simulink model "pmsm_foc"  (R2021a)
settings: Solver=ode23t  StartTime=0.0  StopTime=1  FixedStep=0.000001  RelTol=1e-3
model workspace (MAT data in the model file):
  G1 = -4000
  G2 = 14000
  L = 0.00395
  Rs = 0.485
  Ts = 1e-06
  a = Simulink.Parameter
  a.DataType = 'auto'
  a.Dimensions = [0 0]
undefined symbols (not defined in the file or in its folder): DiscIntNeverNeededParam
libraries: pid_lib x3, spsDCVoltageSourceLib x1, spsGroundLib x1, spsPermanentMagnetSynchronousMachineLib x1, simulink x1, spsUniversalBridgeLib x1, spspowerguiLib x1
settings Model: OrderedModelArguments=off  Creator=SkyLin  LastModifiedBy=SkyLin
settings OptimizationCC: GainParamInheritBuiltInType=on  UseFloatMulNetSlope=on
settings RTWCC: GenCodeOnly=on

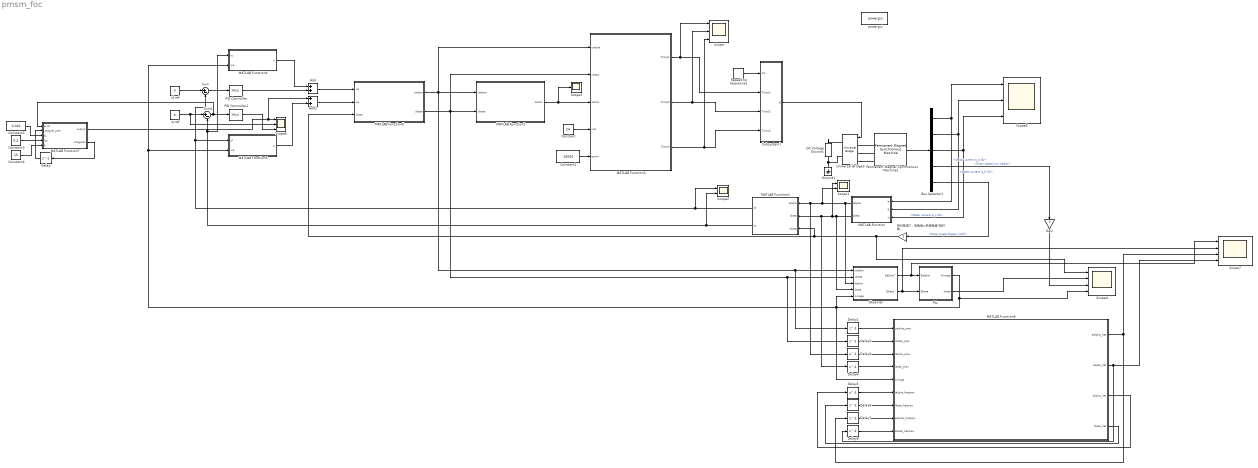
== system pmsm_foc ==
  Add : Sum
  Add1 : Sum
  Bus Selector1 : BusSelector  OutputSignals=Stator current is_a (A),Stator current is_b (A),Stator current is_c (A),Rotor speed wm (rad/s),Rotor angle thetam (rad)
  Constant : Constant  Value=24
  Constant1 : Constant  Value=10000
  Constant2 : Constant  Value=0.001
  Constant3 : Constant  Value=0.4
  Constant4 : Constant  Value=15
  DC Voltage Source1 : spsDCVoltageSourceLib/DC Voltage Source  Amplitude=24  Measurements=None
  Delay{,1..8} (9 alike) : Delay  DelayLength=1
  Gain : Gain  Gain=7
  Ground1 : spsGroundLib/Ground  LConnTagsString=a
  MATLAB Function : MATLAB Function  TreatAsAtomicUnit=on
  MATLAB Function1 : MATLAB Function  TreatAsAtomicUnit=on
  MATLAB Function2 : MATLAB Function  TreatAsAtomicUnit=on
  MATLAB Function3 : MATLAB Function  TreatAsAtomicUnit=on
  MATLAB Function4 : MATLAB Function  TreatAsAtomicUnit=on
  MATLAB Function5 : MATLAB Function  TreatAsAtomicUnit=on
  MATLAB Function6 : MATLAB Function  TreatAsAtomicUnit=on
  MATLAB Function7 : MATLAB Function  TreatAsAtomicUnit=on
  MATLAB Function8 : MATLAB Function  TreatAsAtomicUnit=on
  Observer : Subsystem
  PID Controller : pid_lib/PID Controller  Controller=PI  Form=Parallel  TimeDomain=Discrete-time  UseExternalTs=off  SampleTime=-1  IntegratorMethod=Forward Euler  FilterMethod=Forward Euler  ControllerParametersSource=internal  P=3.05  I=374.17  D=0  UseFilter=on  N=100  TunerSelectOption=Transfer Function Based (PID Tuner App)  InitialConditionSource=internal  InitialConditionForIntegrator=0  InitialConditionForFilter=0  DifferentiatorICPrevScaledInput=0  ExternalReset=none  TrackingMode=off  Kt=1  LimitOutput=on  SatLimitsSource=internal  UpperSaturationLimit=24  LowerSaturationLimit=-24  LinearizeAsGain=on  AntiWindupMode=none  Kb=1  POutMin=[]  POutMax=[]  IOutMin=[]  IOutMax=[]  DOutMin=[]  DOutMax=[]  NOutMin=[]  NOutMax=[]  SumOutMin=[]  SumOutMax=[]  SaturationOutMin=[]  SaturationOutMax=[]  PParamMin=[]  PParamMax=[]  IParamMin=[]  IParamMax=[]  DParamMin=[]  DParamMax=[]  NParamMin=[]  NParamMax=[]  KbParamMin=[]  KbParamMax=[]  KtParamMin=[]  KtParamMax=[]  KbOutMin=[]  KbOutMax=[]  KtOutMin=[]  KtOutMax=[]  IntegratorOutMin=[]  IntegratorOutMax=[]  FilterOutMin=[]  FilterOutMax=[]  SumI1OutMin=[]  SumI1OutMax=[]  SumI2OutMin=[]  SumI2OutMax=[]  SumI3OutMin=[]  SumI3OutMax=[]  SumI4OutMin=[]  SumI4OutMax=[]  SumDOutMin=[]  SumDOutMax=[]  DifferentiatorOutMin=[]  DifferentiatorOutMax=[]  FilterDiffOutCoefMin=[]  FilterDiffOutCoefMax=[]  ReciprocalOutMin=[]  ReciprocalOutMax=[]  SumDenOutMin=[]  SumDenOutMax=[]  SumNumOutMin=[]  SumNumOutMax=[]  DivideOutMin=[]  DivideOutMax=[]  UdiffTsProdOutMin=[]  UdiffTsProdOutMax=[]  NTsProdOutMin=[]  NTsProdOutMax=[]  UintegralTsProdOutMin=[]  UintegralTsProdOutMax=[]  UngainTsProdOutMin=[]  UngainTsProdOutMax=[]  IntegratorContinuousStateAttributes=''  IntegratorStateMustResolveToSignalObject=off  IntegratorRTWStateStorageClass=Auto  FilterContinuousStateAttributes=''  FilterStateMustResolveToSignalObject=off  FilterRTWStateStorageClass=Auto  ParallelPVariant=InternalParameters  IdealPVariant=Disabled  IVariant=InternalParameters  DVariant=Disabled  IntegratorVariant=Discrete  SatVariant=Enabled  AWVariant=Passthrough  PCopyVariant=Disabled  TRVariant=Disabled  FdbkBlocksVariant=Forward  IdealPFdbkVariant=Disabled  SatFdbkVariant=Disabled  DerivativeFilterVariant=Disabled  NVariant=Disabled  NCopyVariant=Disabled_SignalSpec  FilterICVariant=Disabled  IntegratorICVariant=InternalICs  ExternalResetVariant=Disabled  TRSumVariant=Passthrough  SumFdbkVariant=Disabled  SumVariant=Sum_PI  TsampFilterVariant=InternalTs  TsampNgainVariant=Passthrough  TsampIntegralVariant=Passthrough  ExternalSaturationOutDataTypeStr=Inherit: Same as second input
  PID Controller1 : pid_lib/PID Controller  Controller=PI  Form=Parallel  TimeDomain=Discrete-time  UseExternalTs=off  SampleTime=-1  IntegratorMethod=Forward Euler  FilterMethod=Forward Euler  ControllerParametersSource=internal  P=3.15  I=374.17  D=0  UseFilter=on  N=100  TunerSelectOption=Transfer Function Based (PID Tuner App)  InitialConditionSource=internal  InitialConditionForIntegrator=0  InitialConditionForFilter=0  DifferentiatorICPrevScaledInput=0  ExternalReset=none  TrackingMode=off  Kt=1  LimitOutput=on  SatLimitsSource=internal  UpperSaturationLimit=24  LowerSaturationLimit=-24  LinearizeAsGain=on  AntiWindupMode=none  Kb=1  POutMin=[]  POutMax=[]  IOutMin=[]  IOutMax=[]  DOutMin=[]  DOutMax=[]  NOutMin=[]  NOutMax=[]  SumOutMin=[]  SumOutMax=[]  SaturationOutMin=[]  SaturationOutMax=[]  PParamMin=[]  PParamMax=[]  IParamMin=[]  IParamMax=[]  DParamMin=[]  DParamMax=[]  NParamMin=[]  NParamMax=[]  KbParamMin=[]  KbParamMax=[]  KtParamMin=[]  KtParamMax=[]  KbOutMin=[]  KbOutMax=[]  KtOutMin=[]  KtOutMax=[]  IntegratorOutMin=[]  IntegratorOutMax=[]  FilterOutMin=[]  FilterOutMax=[]  SumI1OutMin=[]  SumI1OutMax=[]  SumI2OutMin=[]  SumI2OutMax=[]  SumI3OutMin=[]  SumI3OutMax=[]  SumI4OutMin=[]  SumI4OutMax=[]  SumDOutMin=[]  SumDOutMax=[]  DifferentiatorOutMin=[]  DifferentiatorOutMax=[]  FilterDiffOutCoefMin=[]  FilterDiffOutCoefMax=[]  ReciprocalOutMin=[]  ReciprocalOutMax=[]  SumDenOutMin=[]  SumDenOutMax=[]  SumNumOutMin=[]  SumNumOutMax=[]  DivideOutMin=[]  DivideOutMax=[]  UdiffTsProdOutMin=[]  UdiffTsProdOutMax=[]  NTsProdOutMin=[]  NTsProdOutMax=[]  UintegralTsProdOutMin=[]  UintegralTsProdOutMax=[]  UngainTsProdOutMin=[]  UngainTsProdOutMax=[]  IntegratorContinuousStateAttributes=''  IntegratorStateMustResolveToSignalObject=off  IntegratorRTWStateStorageClass=Auto  FilterContinuousStateAttributes=''  FilterStateMustResolveToSignalObject=off  FilterRTWStateStorageClass=Auto  ParallelPVariant=InternalParameters  IdealPVariant=Disabled  IVariant=InternalParameters  DVariant=Disabled  IntegratorVariant=Discrete  SatVariant=Enabled  AWVariant=Passthrough  PCopyVariant=Disabled  TRVariant=Disabled  FdbkBlocksVariant=Forward  IdealPFdbkVariant=Disabled  SatFdbkVariant=Disabled  DerivativeFilterVariant=Disabled  NVariant=Disabled  NCopyVariant=Disabled_SignalSpec  FilterICVariant=Disabled  IntegratorICVariant=InternalICs  ExternalResetVariant=Disabled  TRSumVariant=Passthrough  SumFdbkVariant=Disabled  SumVariant=Sum_PI  TsampFilterVariant=InternalTs  TsampNgainVariant=Passthrough  TsampIntegralVariant=Passthrough  ExternalSaturationOutDataTypeStr=Inherit: Same as second input
  PLL : Subsystem
  Permanent Magnet Synchronous Machine1 : spsPermanentMagnetSynchronousMachineLib/Permanent Magnet Synchronous Machine  NbPhases=3  FluxDistribution=Sinusoidal  RotorType=Round  MechanicalLoad=Torque Tm  PresetModel=No  ShowDetailedParameters=on  MeasurementBus=off  Resistance=0.485  Inductance=8.5e-3  dqInductances=[8.5e-3,8.5e-3]  La=0.00395  MachineConstant=Flux linkage established by magnets (V.s)  Flux=0.0041087  VoltageCst=5.2167  TorqueCst=0.043141  Flat=120  Mechanical=[0.00007 0.04924 7 0]  PolePairs=4  InitialConditions=[0,0, 0,0]  InitialConditions5ph=[0 0 0 0 0 0]  RefAngle=Aligned with phase A axis (original Park)  IterativeDiscreteModel=Trapezoidal non iterative  TsBlock=-1  TsPowergui=0
  Repeating Sequence1 : simulink/Sources/Repeating Sequence  rep_seq_t=[0 0.0001 0.0002]  rep_seq_y=[0 10000 0]
  Scope : Scope  NumInputPorts=3
  Scope1 : Scope  NumInputPorts=2
  Scope2 : Scope  NumInputPorts=2
  Scope3 : Scope
  Scope4 : Scope  NumInputPorts=4
  Scope5 : Scope  NumInputPorts=3
  Scope6 : Scope  NumInputPorts=3
  Scope7 : Scope  NumInputPorts=4
  Subsystem1 : Subsystem
  Sum : Sum  Inputs=|+-
  Sum1 : Sum  Inputs=|+-
  Universal Bridge3 : spsUniversalBridgeLib/Universal Bridge  Arms=3  SnubberResistance=1e5  SnubberCapacitance=inf  Device=MOSFET / Diodes  Ron=1e-3  Lon=0  ForwardVoltages="[  0  0  ]"  ForwardVoltage=0  GTOparameters=[ 10e-6 , 20e-6 ]  IGBTparameters=[ 1e-6 , 2e-6 ]  Measurements=None  Measurements_2=None  converterType=Rectifier
  id ref : Constant  Value=0
  iq ref : Constant  Value=4
  powergui : spspowerguiLib/powergui  Priority=1  SimulationMode=Discrete  SampleTime=10E-6  frequency=60  Iterations=50  frequencyindice=0  Pbase=100e6  ErrMax=1e-4  UnitsV=kV  UnitsW=MW  buscounter=0  FunctionMessages=off  echomessages=off  EnableUseOfTLC=off  CurrentSourceSwitches=off  DisableSnubberDevices=off  DisableRonSwitches=off  DisableVfSwitches=off  DisplayEquations=off  AutomaticDiscreteSolvers=off  SolverType=Tustin/Backward Euler (TBE)  Interpol=off  ExternalGateDelay=off  methode=off  Ts=100  x0status=blocks  SPID=on  SwTol=0  HookPort=off  NonlinearTolerance=1e-4  nMaxIteration=100  ContinueOnMaxIteration=off  RestoreLinks=warning  ResistiveCurrentMeasurement=off  Frange=[0:2:500]  Ylog=off  Xlog=on  ShowGrid=off  save=off  variable=ZData  structure=0  ZoomFFT=off  StartTime=0.0  cycles=1  DisplayStyle=1  fundamental=60  FreqAxis=off  MaxFrequency=1000  frequencyindicesteady=1  RmsSteady=1  display=off
  极对数是7，电角度=机械角度*极对数 : Gain  Gain=7
  wires:
  Repeating Sequence1/1 -> Subsystem1/1(In1)
  Subsystem1/1(g) -> Universal Bridge3/1
  Permanent Magnet Synchronous Machine1/1 -> Bus Selector1/1
  Bus Selector1/1 -> MATLAB Function/1(ia), Scope5/1  "<Stator current is_a (A)>"
  Bus Selector1/2 -> Scope5/2, MATLAB Function/2(ib)  "<Stator current is_b (A)>"
  Bus Selector1/3 -> Scope5/3, MATLAB Function/3(ic)  "<Stator current is_c (A)>"
  极对数是7，电角度=机械角度*极对数/1 -> Scope4/1, MATLAB Function1/3(theta), MATLAB Function6/3(theta)
  MATLAB Function/1(ialpha) -> Observer/3(ialpha), Scope1/2, Delay3/1, MATLAB Function1/1(ialpha)
  MATLAB Function/2(ibeta) -> Scope1/1, Delay4/1, MATLAB Function1/2(ibeta), Observer/4(ibeta)
  MATLAB Function6/1(ualpha) -> MATLAB Function3/1(ualpha), Delay1/1, Observer/1(ualpha), MATLAB Function2/1(ualpha)
  MATLAB Function6/2(ubeta) -> MATLAB Function3/2(ubeta), MATLAB Function2/2(ubeta), Delay2/1, Observer/2(ubeta)
  MATLAB Function2/1(sector) -> Scope3/1, MATLAB Function3/3(sector)
  Constant/1 -> MATLAB Function3/4(udc)
  Constant1/1 -> MATLAB Function3/5(tpwm)
  MATLAB Function3/1(Tcmp1) -> Scope/1, Subsystem1/2(Tcmp1)
  MATLAB Function3/2(Tcmp2) -> Scope/2, Subsystem1/3(Tcmp2)
  MATLAB Function3/3(Tcmp3) -> Scope/3, Subsystem1/4(Tcmp3)
  Bus Selector1/5 -> 极对数是7，电角度=机械角度*极对数/1  "<Rotor angle thetam (rad)>"
  Observer/1(Ealpha^) -> Scope7/1, PLL/1(Ealpha)
  Observer/2(Ebeta^) -> PLL/2(Ebeta), Scope7/2
  id ref/1 -> Sum/1
  MATLAB Function1/1(id) -> Scope2/1, MATLAB Function5/1(id), Sum/2
  iq ref/1 -> Scope6/2, Sum1/1
  Sum/1 -> PID Controller/1
  Sum1/1 -> MATLAB Function7/1(error), PID Controller1/1
  MATLAB Function1/2(iq) -> Scope2/2, MATLAB Function4/1(iq), Sum1/2
  Bus Selector1/4 -> Gain/1  "<Rotor speed wm (rad/s)>"
  MATLAB Function4/1(y) -> Add/1
  PID Controller/1 -> Add/2
  Add/1 -> MATLAB Function6/1(ud)
  Add1/1 -> MATLAB Function6/2(uq)
  PID Controller1/1 -> Scope6/3
  MATLAB Function5/1(y) -> Add1/2
  PLL/2(theta) -> Scope4/2
  Gain/1 -> Scope4/3
  PLL/1(Omega) -> MATLAB Function8/5(omega), MATLAB Function4/2(we), MATLAB Function5/2(we), Observer/5(omega), Scope4/4
  Constant2/1 -> MATLAB Function7/3(ts)
  MATLAB Function7/1(output) -> Add1/1, Scope6/1
  MATLAB Function7/2(integeral) -> Delay/1
  Delay/1 -> MATLAB Function7/2(integral_prev)
  Constant3/1 -> MATLAB Function7/4(kp)
  Constant4/1 -> MATLAB Function7/5(ki)
  Delay1/1 -> MATLAB Function8/1(ualpha_prev)
  Delay2/1 -> MATLAB Function8/2(ubeta_prev)
  Delay3/1 -> MATLAB Function8/3(ialpha_prev)
  Delay4/1 -> MATLAB Function8/4(ibeta_prev)
  Delay5/1 -> MATLAB Function8/6(ialpha_hatprev)
  Delay6/1 -> MATLAB Function8/7(ibeta_hatprev)
  Delay7/1 -> MATLAB Function8/8(ealpha_hatprev)
  Delay8/1 -> MATLAB Function8/9(ebeta_hatprev)
  MATLAB Function8/3(ialpha_hat) -> Delay5/1
  MATLAB Function8/4(ibeta_hat) -> Delay6/1
  MATLAB Function8/2(ebeta_hat) -> Delay8/1, Scope7/4
  MATLAB Function8/1(ealpha_hat) -> Delay7/1, Scope7/3
  connections:
  DC Voltage Source1/RConn1 -- Universal Bridge3/RConn1
  Permanent Magnet Synchronous Machine1/LConn1 -- Universal Bridge3/LConn1
  Universal Bridge3/LConn2 -- Permanent Magnet Synchronous Machine1/LConn2
  Universal Bridge3/LConn3 -- Permanent Magnet Synchronous Machine1/LConn3
  DC Voltage Source1/LConn1 -- Ground1/LConn1 -- Universal Bridge3/RConn2

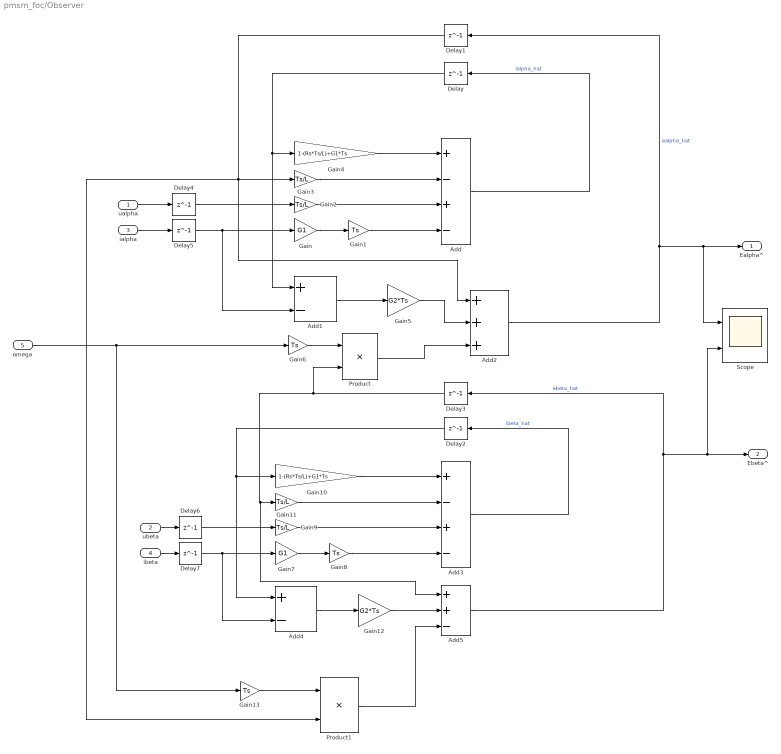
== system pmsm_foc/Observer ==
  ualpha : Inport
  ubeta : Inport  Port=2
  ialpha : Inport  Port=3
  ibeta : Inport  Port=4
  omega : Inport  Port=5
  Add : Sum  Inputs=+-+-
  Add1 : Sum  Inputs=+-
  Add2 : Sum  Inputs=+++
  Add3 : Sum  Inputs=+-+-
  Add4 : Sum  Inputs=+-
  Add5 : Sum  Inputs=++-
  Delay{,1..7} (8 alike) : Delay  DelayLength=1
  Gain : Gain  Gain=G1
  Gain{1,6,8,13} (4 alike) : Gain  Gain=Ts
  Gain10 : Gain  Gain=1-(Rs*Ts/L)+G1*Ts
  Gain{2..3,9,11} (4 alike) : Gain  Gain=Ts/L
  Gain12 : Gain  Gain=G2*Ts
  Gain4 : Gain  Gain=1-(Rs*Ts/L)+G1*Ts
  Gain5 : Gain  Gain=G2*Ts
  Gain7 : Gain  Gain=G1
  Product : Product
  Product1 : Product
  Scope : Scope  NumInputPorts=2
  Ealpha^ : Outport
  Ebeta^ : Outport  Port=2
  wires:
  Add/1 -> Delay/1  "ialpha_hat"
  ialpha/1 -> Delay5/1
  Gain/1 -> Gain1/1
  Gain1/1 -> Add/4
  ualpha/1 -> Delay4/1
  Gain2/1 -> Add/3
  Gain3/1 -> Add/2
  Gain4/1 -> Add/1
  Delay/1 -> Add1/1, Gain4/1
  Add1/1 -> Gain5/1
  Gain5/1 -> Add2/2
  Add2/1 -> Scope/1, Ealpha^/1, Delay1/1  "ealpha_hat"
  Delay1/1 -> Gain3/1, Product1/2, Add2/1
  Gain6/1 -> Product/1
  Product/1 -> Add2/3
  ibeta/1 -> Delay7/1
  Gain7/1 -> Gain8/1
  Gain8/1 -> Add3/4
  ubeta/1 -> Delay6/1
  Gain9/1 -> Add3/3
  Add3/1 -> Delay2/1  "ibeta_hat"
  Delay2/1 -> Gain10/1, Add4/1
  Gain10/1 -> Add3/1
  Gain11/1 -> Add3/2
  Add4/1 -> Gain12/1
  Gain12/1 -> Add5/2
  Add5/1 -> Scope/2, Ebeta^/1, Delay3/1  "ebeta_hat"
  Delay3/1 -> Product/2, Add5/1, Gain11/1
  Gain13/1 -> Product1/1
  omega/1 -> Gain13/1, Gain6/1
  Product1/1 -> Add5/3
  Delay4/1 -> Gain2/1
  Delay5/1 -> Add1/2, Gain/1
  Delay6/1 -> Gain9/1
  Delay7/1 -> Add4/2, Gain7/1

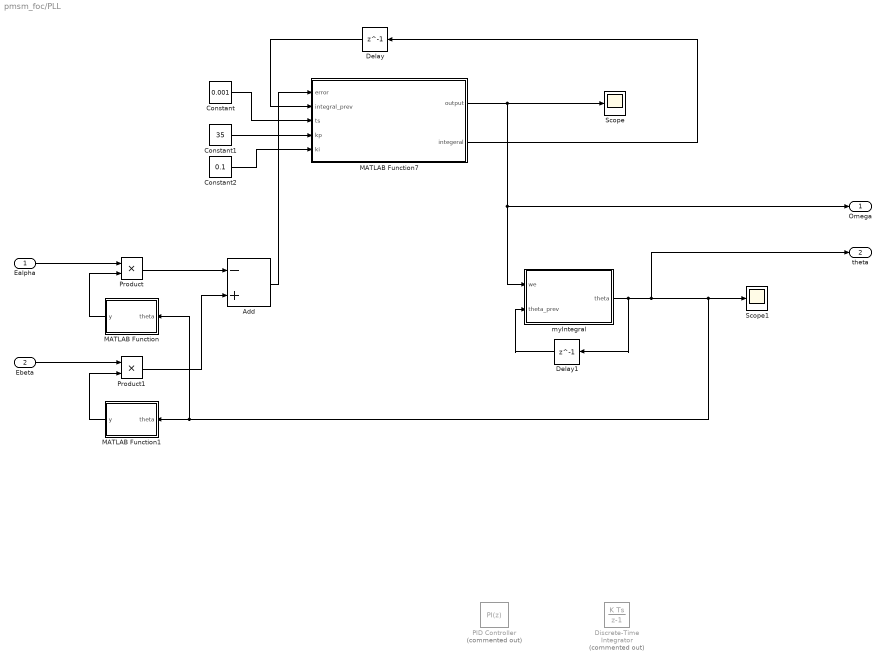
== system pmsm_foc/PLL ==
  Ealpha : Inport
  Ebeta : Inport  Port=2
  Add : Sum  Inputs=-+
  Constant : Constant  Value=0.001
  Constant1 : Constant  Value=35
  Constant2 : Constant  Value=0.1
  Delay : Delay  DelayLength=1
  Delay1 : Delay  DelayLength=1
  Discrete-Time Integrator : DiscreteIntegrator  Commented=on  SampleTime=-1  ICPrevOutput=DiscIntNeverNeededParam  ICPrevScaledInput=DiscIntNeverNeededParam
  MATLAB Function : MATLAB Function  TreatAsAtomicUnit=on
  MATLAB Function1 : MATLAB Function  TreatAsAtomicUnit=on
  MATLAB Function7 : MATLAB Function  TreatAsAtomicUnit=on
  PID Controller : pid_lib/PID Controller  Commented=on  Controller=PI  Form=Parallel  TimeDomain=Discrete-time  UseExternalTs=off  SampleTime=-1  IntegratorMethod=Forward Euler  FilterMethod=Forward Euler  ControllerParametersSource=internal  P=35  I=0.5  D=0  UseFilter=on  N=100  TunerSelectOption=Transfer Function Based (PID Tuner App)  InitialConditionSource=internal  InitialConditionForIntegrator=0  InitialConditionForFilter=0  DifferentiatorICPrevScaledInput=0  ExternalReset=none  TrackingMode=off  Kt=1  LimitOutput=off  SatLimitsSource=internal  UpperSaturationLimit=inf  LowerSaturationLimit=0  LinearizeAsGain=on  AntiWindupMode=none  Kb=1  POutMin=[]  POutMax=[]  IOutMin=[]  IOutMax=[]  DOutMin=[]  DOutMax=[]  NOutMin=[]  NOutMax=[]  SumOutMin=[]  SumOutMax=[]  SaturationOutMin=[]  SaturationOutMax=[]  PParamMin=[]  PParamMax=[]  IParamMin=[]  IParamMax=[]  DParamMin=[]  DParamMax=[]  NParamMin=[]  NParamMax=[]  KbParamMin=[]  KbParamMax=[]  KtParamMin=[]  KtParamMax=[]  KbOutMin=[]  KbOutMax=[]  KtOutMin=[]  KtOutMax=[]  IntegratorOutMin=[]  IntegratorOutMax=[]  FilterOutMin=[]  FilterOutMax=[]  SumI1OutMin=[]  SumI1OutMax=[]  SumI2OutMin=[]  SumI2OutMax=[]  SumI3OutMin=[]  SumI3OutMax=[]  SumI4OutMin=[]  SumI4OutMax=[]  SumDOutMin=[]  SumDOutMax=[]  DifferentiatorOutMin=[]  DifferentiatorOutMax=[]  FilterDiffOutCoefMin=[]  FilterDiffOutCoefMax=[]  ReciprocalOutMin=[]  ReciprocalOutMax=[]  SumDenOutMin=[]  SumDenOutMax=[]  SumNumOutMin=[]  SumNumOutMax=[]  DivideOutMin=[]  DivideOutMax=[]  UdiffTsProdOutMin=[]  UdiffTsProdOutMax=[]  NTsProdOutMin=[]  NTsProdOutMax=[]  UintegralTsProdOutMin=[]  UintegralTsProdOutMax=[]  UngainTsProdOutMin=[]  UngainTsProdOutMax=[]  IntegratorContinuousStateAttributes=''  IntegratorStateMustResolveToSignalObject=off  IntegratorRTWStateStorageClass=Auto  FilterContinuousStateAttributes=''  FilterStateMustResolveToSignalObject=off  FilterRTWStateStorageClass=Auto  ParallelPVariant=InternalParameters  IdealPVariant=Disabled  IVariant=InternalParameters  DVariant=Disabled  IntegratorVariant=Discrete  SatVariant=Disabled  AWVariant=Passthrough  PCopyVariant=Disabled  TRVariant=Disabled  FdbkBlocksVariant=Forward  IdealPFdbkVariant=Disabled  SatFdbkVariant=Disabled  DerivativeFilterVariant=Disabled  NVariant=Disabled  NCopyVariant=Disabled_SignalSpec  FilterICVariant=Disabled  IntegratorICVariant=InternalICs  ExternalResetVariant=Disabled  TRSumVariant=Passthrough  SumFdbkVariant=Disabled  SumVariant=Sum_PI  TsampFilterVariant=InternalTs  TsampNgainVariant=Passthrough  TsampIntegralVariant=Passthrough  ExternalSaturationOutDataTypeStr=Inherit: Same as second input
  Product : Product
  Product1 : Product
  Scope : Scope
  Scope1 : Scope
  myIntegral : MATLAB Function  TreatAsAtomicUnit=on
  Omega : Outport
  theta : Outport  Port=2
  wires:
  Ealpha/1 -> Product/1
  MATLAB Function/1(y) -> Product/2
  Ebeta/1 -> Product1/1
  MATLAB Function1/1(y) -> Product1/2
  Product/1 -> Add/1
  Product1/1 -> Add/2
  MATLAB Function7/2(integeral) -> Delay/1
  Delay/1 -> MATLAB Function7/2(integral_prev)
  MATLAB Function7/1(output) -> myIntegral/1(we), Omega/1, Scope/1
  Constant/1 -> MATLAB Function7/3(ts)
  Constant2/1 -> MATLAB Function7/5(ki)
  Constant1/1 -> MATLAB Function7/4(kp)
  myIntegral/1(theta) -> Delay1/1, theta/1, MATLAB Function/1(theta), MATLAB Function1/1(theta), Scope1/1
  Delay1/1 -> myIntegral/2(theta_prev)
  Add/1 -> MATLAB Function7/1(error)

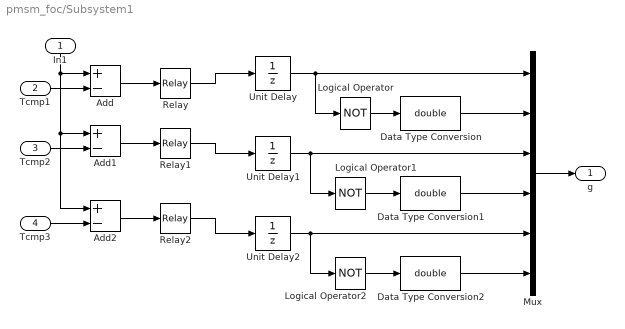
== system pmsm_foc/Subsystem1 ==
  In1 : Inport
  Tcmp1 : Inport  Port=2
  Tcmp2 : Inport  Port=3
  Tcmp3 : Inport  Port=4
  Add : Sum  Inputs=+-
  Add1 : Sum  Inputs=+-
  Add2 : Sum  Inputs=+-
  Data Type Conversion : DataTypeConversion  OutDataTypeStr=double
  Data Type Conversion1 : DataTypeConversion  OutDataTypeStr=double
  Data Type Conversion2 : DataTypeConversion  OutDataTypeStr=double
  Logical Operator : Logic  Operator=NOT  AllPortsSameDT=off  OutDataTypeStr=boolean
  Logical Operator1 : Logic  Operator=NOT  AllPortsSameDT=off  OutDataTypeStr=boolean
  Logical Operator2 : Logic  Operator=NOT  AllPortsSameDT=off  OutDataTypeStr=boolean
  Mux : Mux  Inputs=6
  Relay : Relay  OffSwitchValue=-eps
  Relay1 : Relay  OffSwitchValue=-eps
  Relay2 : Relay  OffSwitchValue=-eps
  Unit Delay : UnitDelay  SampleTime=-1  HasFrameUpgradeWarning=on
  Unit Delay1 : UnitDelay  SampleTime=-1  HasFrameUpgradeWarning=on
  Unit Delay2 : UnitDelay  SampleTime=-1  HasFrameUpgradeWarning=on
  g : Outport  VectorParamsAs1DForOutWhenUnconnected=off
  wires:
  Tcmp3/1 -> Add2/2
  Tcmp2/1 -> Add1/2
  Tcmp1/1 -> Add/2
  Relay2/1 -> Unit Delay2/1
  Relay1/1 -> Unit Delay1/1
  Relay/1 -> Unit Delay/1
  Unit Delay2/1 -> Mux/5, Logical Operator2/1
  Unit Delay1/1 -> Mux/3, Logical Operator1/1
  Unit Delay/1 -> Logical Operator/1, Mux/1
  Mux/1 -> g/1
  Data Type Conversion/1 -> Mux/2
  Data Type Conversion1/1 -> Mux/4
  Data Type Conversion2/1 -> Mux/6
  Logical Operator2/1 -> Data Type Conversion2/1
  Logical Operator1/1 -> Data Type Conversion1/1
  Logical Operator/1 -> Data Type Conversion/1
  Add1/1 -> Relay1/1
  Add2/1 -> Relay2/1
  Add/1 -> Relay/1
  In1/1 -> Add/1, Add2/1, Add1/1

== matlab function pmsm_foc/MATLAB Function8 ==
  data: ealpha_hat output; ebeta_hat output; ualpha_prev input; ialpha_hat output; ubeta_prev input; ialpha_prev input; ibeta_prev input; omega input; ialpha_hatprev input; ibeta_hatprev input; ealpha_hatprev input; ebeta_hatprev input; ibeta_hat output
function [ealpha_hat,ebeta_hat,ialpha_hat,ibeta_hat] = luenberger(ualpha_prev,ubeta_prev,ialpha_prev,ibeta_prev,omega,ialpha_hatprev,ibeta_hatprev,ealpha_hatprev,ebeta_hatprev)

Ts=1e-6;
G1=-4000;
G2=14000;
L=0.00395;
Rs=0.485;


ialpha_hat=(1-Rs*Ts/L+G1*Ts)*ialpha_hatprev-(Ts/L)*ealpha_hatprev+(Ts/L)*ualpha_prev+G1*Ts*(-ialpha_prev);
ibeta_hat=(1-Rs*Ts/L+G1*Ts)*ibeta_hatprev-(Ts/L)*ebeta_hatprev+(Ts/L)*ubeta_prev+G1*Ts*(-ibeta_prev);
ealpha_hat=ealpha_hatprev+omega*Ts*ebeta_hatprev+G2*Ts*(ialpha_hatprev-ialpha_prev);
ebeta_hat=ebeta_hatprev-omega*Ts*ealpha_hat+G2*Ts*(ibeta_hatprev-ibeta_prev);


end

== matlab function pmsm_foc/PLL/MATLAB Function7 ==
  data: error input; output output; integral_prev input; integeral output; ts input; kp input; ki input
function [output,integeral] = PI_CTRL(error,integral_prev,ts,kp,ki)


p_val=kp*error;
i_val=integral_prev+ki*ts*error;

output=p_val+i_val;
integeral=i_val;


end

== matlab function pmsm_foc/PLL/myIntegral ==
  data: we input; theta output; theta_prev input
function theta = fcn(we,theta_prev)

ts=1e-5;

theta=theta_prev+we*ts;

end

== matlab function pmsm_foc/MATLAB Function1 ==
  data: ialpha input; id output; ibeta input; theta input; iq output
function [id,iq] = Park(ialpha,ibeta,theta)
id = ialpha*cos(theta)+ibeta*sin(theta);
iq = -ialpha*sin(theta)+ibeta*cos(theta);

== matlab function pmsm_foc/MATLAB Function ==
  data: ia input; ialpha output; ib input; ic input; ibeta output
function [ialpha,ibeta] = Clark(ia,ib,ic)
ialpha = ia*2/3-(ib+ic)/3;
ibeta = (ib-ic)*sqrt(3)/3;

== matlab function pmsm_foc/MATLAB Function2 ==
  data: ualpha input; sector output; ubeta input
function sector = JudgeSector(ualpha,ubeta)

sector=single(0); %优先初始化

uref1=ubeta;
uref2=(sqrt(3)/2)*ualpha-(1/2)*ubeta;
uref3=(-sqrt(3)/2)*ualpha-(1/2)*ubeta;

if uref1>0
    sector=single(1);
end

if uref2>0
    sector=sector+single(2);
end

if uref3>0
    sector=sector+single(4);
end


end

== matlab function pmsm_foc/MATLAB Function3 ==
  data: ualpha input; ubeta input; sector input; Tcmp1 output; udc input; tpwm input; Tcmp2 output; Tcmp3 output
function [Tcmp1,Tcmp2,Tcmp3] = SVPWM(ualpha,ubeta,sector,udc,tpwm)

Tcmp1=double(0);
Tcmp2=double(0);
Tcmp3=double(0);

X = sqrt(3)*ubeta*tpwm/udc;
Y = tpwm/udc*(3/2*ualpha+sqrt(3)/2*ubeta);
Z = tpwm/udc*(-3/2*ualpha+sqrt(3)/2*ubeta);	

switch (sector)   
    case 1
        T1 = Z; T2 = Y; 
	case 2
        T1 = Y; T2 = -X; 
	case 3
        T1 = -Z; T2 = X; 
	case 4
        T1 = -X; T2 = Z;
	case 5
        T1 = X; T2 = -Y;
    otherwise
        T1 = -Y; T2 = -Z;
end

temp=T1+T2;

if T1+T2 > tpwm
    T1 = T1/temp;
    T2 = T2/temp;
else
    T1 = T1;
    T2 = T2;
end
ta = (tpwm-(T1+T2))/4.0;
tb = ta+T1/2;
tc = tb+T2/2;

%=CCR计算=%

switch (sector)
    case 1 
        Tcmp1=tb;
        Tcmp2=ta;
        Tcmp3=tc; 
        
    case 2 
        Tcmp1=ta;
        Tcmp2=tc;
        Tcmp3=tb; 
       
    case 3 
        Tcmp1=ta;
        Tcmp2=tb;
        Tcmp3=tc; 
        
    case 4 
        Tcmp1=tc;
        Tcmp2=tb;
        Tcmp3=ta;
        
    case 5 
        Tcmp1=tc;
        Tcmp2=ta;
        Tcmp3=tb;
        
   case 6
       Tcmp1=tb;
       Tcmp2=tc;
       Tcmp3=ta;
end

end

== matlab function pmsm_foc/PLL/MATLAB Function ==
  data: theta input; y output
function y = Sin(theta)

y=sin(theta);
end

== matlab function pmsm_foc/PLL/MATLAB Function1 ==
  data: theta input; y output
function y = Cos(theta)

y=cos(theta);
end

== matlab function pmsm_foc/MATLAB Function4 ==
  data: iq input; y output; we input
function y = DForward(iq,we)

y = -we*iq*0.0041087;
end

== matlab function pmsm_foc/MATLAB Function5 ==
  data: id input; y output; we input
function y = QForward(id,we)

y = we*(0.0041087+0.00395*id);
end

== matlab function pmsm_foc/MATLAB Function6 ==
  data: ud input; ualpha output; uq input; theta input; ubeta output
function [ualpha,ubeta] = AntiPark(ud, uq, theta)
ualpha=ud*cos(theta)-uq*sin(theta)
ubeta=ud*sin(theta)+uq*cos(theta)

== matlab function pmsm_foc/MATLAB Function7 ==
  data: error input; output output; integral_prev input; integeral output; ts input; kp input; ki input
function [output,integeral] = PI_CTRL(error,integral_prev,ts,kp,ki)


p_val=kp*error;
i_val=integral_prev+ki*ts*error;

output=p_val+i_val;
integeral=i_val;

%=限幅=%
if output>10
    output=10;
elseif output<-10
    output=-10;
end


end
